simulink model "quadcopter_alt_simple"  (R2021a)
settings: Solver=VariableStepAuto  StartTime=0.0  StopTime=10.0  RelTol=1e-3
undefined symbols (not defined in the file): DiscIntNeverNeededParam
settings Model: Creator=turkcuoglu  LastModifiedBy=turkcuoglu

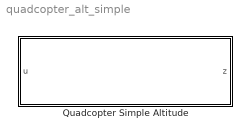
== system quadcopter_alt_simple ==
  Quadcopter Simple Altitude : Subsystem  mask{g=9.807, m=0.028, SampleTime=-1}
      mask prompts: g "Gravity constant g"; m "Mass of quadrotor"; SampleTime "Simulink:blkprm_prompts:AllBlksSampleTime"
      mask TypeOptions SampleTime: u/SampleTime
      mask DialogControl SampleTime Prompt: Sample time (-1 for inherited):

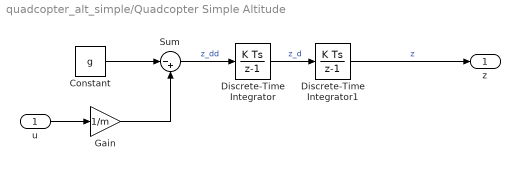
== system quadcopter_alt_simple/Quadcopter Simple Altitude ==
  u : Inport  SampleTime=SampleTime
  Constant : Constant  Value=g  SampleTime=-1
  Discrete-Time Integrator : DiscreteIntegrator  SampleTime=-1  ICPrevOutput=DiscIntNeverNeededParam  ICPrevScaledInput=DiscIntNeverNeededParam
  Discrete-Time Integrator1 : DiscreteIntegrator  SampleTime=-1  LimitOutput=on  LowerSaturationLimit=0  ICPrevOutput=DiscIntNeverNeededParam  ICPrevScaledInput=DiscIntNeverNeededParam
  Gain : Gain  Gain=1/m
  Sum : Sum  Inputs=|-+
  z : Outport
  wires:
  Sum/1 -> Discrete-Time Integrator/1  "z_dd"
  Discrete-Time Integrator1/1 -> z/1  "z"
  Constant/1 -> Sum/1
  Gain/1 -> Sum/2
  u/1 -> Gain/1
  Discrete-Time Integrator/1 -> Discrete-Time Integrator1/1  "z_d"
